simulink model "model_observer_controller_noise"  (R2024a)
settings: Solver=FixedStepAuto  StartTime=0.0  StopTime=10.0  RelTol=1e-3
undefined symbols (not defined in the file): A, B, C, D, K, L, x0, x_hat0
settings Model: Creator=anton  LastModifiedBy=anton

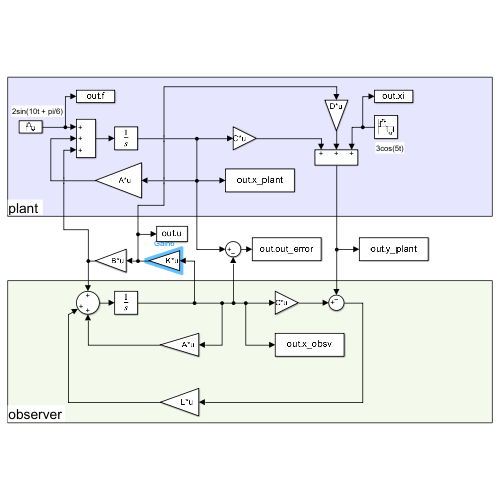
[thumbnail: Simulink's stored preview of the top-level diagram]
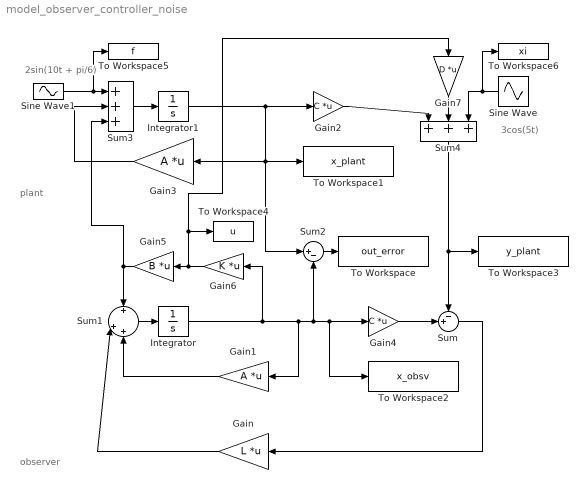
== system model_observer_controller_noise ==
  note: 2sin(10t + pi/6)
  note: 3cos(5t)
  note: plant
  note: observer
  Gain : Gain  Gain=L  Multiplication=Matrix(K*u)
  Gain1 : Gain  Gain=A  Multiplication=Matrix(K*u)
  Gain2 : Gain  Gain=C  Multiplication=Matrix(K*u)
  Gain3 : Gain  Gain=A  Multiplication=Matrix(K*u)
  Gain4 : Gain  Gain=C  Multiplication=Matrix(K*u)
  Gain5 : Gain  Gain=B  Multiplication=Matrix(K*u)
  Gain6 : Gain  Gain=K  Multiplication=Matrix(K*u)
  Gain7 : Gain  Gain=D  Multiplication=Matrix(K*u)
  Integrator : Integrator  InitialCondition=x_hat0
  Integrator1 : Integrator  InitialCondition=x0
  Sine Wave : Sin  Amplitude=3  Frequency=5  Phase=pi/2  SampleTime=0.0001
  Sine Wave1 : Sin  Amplitude=2  Frequency=10  Phase=pi/6  SampleTime=0.0001
  Sum : Sum  Inputs=-+|
  Sum1 : Sum  Inputs=+|++
  Sum2 : Sum  Inputs=|+-
  Sum3 : Sum  Inputs=+++
  Sum4 : Sum  Inputs=+++
  To Workspace : ToWorkspace  VariableName=out_error  SaveFormat=Timeseries  SampleTime=-1
  To Workspace1 : ToWorkspace  VariableName=x_plant  SaveFormat=Timeseries  SampleTime=-1
  To Workspace2 : ToWorkspace  VariableName=x_obsv  SaveFormat=Timeseries  SampleTime=-1
  To Workspace3 : ToWorkspace  VariableName=y_plant  SaveFormat=Timeseries  SampleTime=-1
  To Workspace4 : ToWorkspace  VariableName=u  SaveFormat=Timeseries  SampleTime=-1
  To Workspace5 : ToWorkspace  VariableName=f  SaveFormat=Timeseries  SampleTime=-1
  To Workspace6 : ToWorkspace  VariableName=xi  SaveFormat=Timeseries  SampleTime=-1
  wires:
  Gain5/1 -> Sum3/3, Sum1/1
  Gain4/1 -> Sum/2
  Sum3/1 -> Integrator1/1
  Sum2/1 -> To Workspace/1
  Sum1/1 -> Integrator/1
  Integrator/1 -> Gain6/1, Gain1/1, Sum2/2, To Workspace2/1, Gain4/1
  Sum/1 -> Gain/1
  Integrator1/1 -> Sum2/1, To Workspace1/1, Gain3/1, Gain2/1
  Gain/1 -> Sum1/2
  Gain1/1 -> Sum1/3
  Gain6/1 -> Gain7/1, To Workspace4/1, Gain5/1
  Gain7/1 -> Sum4/2
  Gain2/1 -> Sum4/1
  Sum4/1 -> To Workspace3/1, Sum/1
  Sine Wave/1 -> To Workspace6/1, Sum4/3
  Gain3/1 -> Sum3/2
  Sine Wave1/1 -> To Workspace5/1, Sum3/1
